simulink model "CompleteCavityModel"  (R2022b)
settings: Solver=VariableStepAuto  StartTime=0.0  StopTime=100  RelTol=1e-3
model workspace (MAT data in the model file):
  KL1 = Simulink.Parameter
  KL1.Value = 0.4
  KL1.DataType = 'auto'
  KL1.Complexity = 'real'
  KL1.Dimensions = [1 1]
  KL2 = Simulink.Parameter
  KL2.Value = 0.3
  KL2.DataType = 'auto'
  KL2.Complexity = 'real'
  KL2.Dimensions = [1 1]
  KL3 = Simulink.Parameter
  KL3.Value = 0.2
  KL3.DataType = 'auto'
  KL3.Complexity = 'real'
  KL3.Dimensions = [1 1]
  QL = Simulink.Parameter
  QL.Value = 960000
  QL.DataType = 'auto'
  QL.Complexity = 'real'
  QL.Dimensions = [1 1]
  Q_k1 = Simulink.Parameter
  Q_k1.Value = 100
  Q_k1.DataType = 'auto'
  Q_k1.Complexity = 'real'
  Q_k1.Dimensions = [1 1]
  Q_k2 = Simulink.Parameter
  Q_k2.Value = 100
  Q_k2.DataType = 'auto'
  Q_k2.Complexity = 'real'
  Q_k2.Dimensions = [1 1]
  Q_k3 = Simulink.Parameter
  Q_k3.Value = 100
  Q_k3.DataType = 'auto'
  Q_k3.Complexity = 'real'
  Q_k3.Dimensions = [1 1]
  RL = Simulink.Parameter
  RL.Value = Simulink.data.Expression
  RL.Value.ExpressionString = "QL*RQ"
  RL.DataType = 'auto'
  RL.Complexity = 'real'
  RL.Dimensions = -1
  RQ = Simulink.Parameter
  RQ.Value = 310
  RQ.DataType = 'auto'
  RQ.Complexity = 'real'
  RQ.Dimensions = [1 1]
  Ts = Simulink.Parameter
  Ts.Value = 1e-10
  Ts.DataType = 'auto'
  Ts.Complexity = 'real'
  Ts.Dimensions = [1 1]
  a0 = Simulink.Parameter
  a0.Value = 1
  a0.DataType = 'auto'
  a0.Complexity = 'real'
  a0.Dimensions = [1 1]
  a1 = Simulink.Parameter
  a1.Value = -2
  a1.DataType = 'auto'
  a1.Complexity = 'real'
  a1.Dimensions = [1 1]
  a2 = Simulink.Parameter
  a2.Value = 1
  a2.DataType = 'auto'
  a2.Complexity = 'real'
  a2.Dimensions = [1 1]
  b0 = Simulink.Parameter
  b0.Value = -2.18e-09
  b0.DataType = 'auto'
  b0.Complexity = 'real'
  b0.Dimensions = [1 1]
  b1 = Simulink.Parameter
  b1.Value = -4.36e-09
  b1.DataType = 'auto'
  b1.Complexity = 'real'
  b1.Dimensions = [1 1]
  b2 = Simulink.Parameter
  b2.Value = -2.18e-09
  b2.DataType = 'auto'
  b2.Complexity = 'real'
  b2.Dimensions = [1 1]
  f0 = Simulink.Parameter
  f0.Value = 648000000
  f0.DataType = 'auto'
  f0.Complexity = 'real'
  f0.Dimensions = [1 1]
  f_k1 = Simulink.Parameter
  f_k1.Value = 235
  f_k1.DataType = 'auto'
  f_k1.Complexity = 'real'
  f_k1.Dimensions = [1 1]
  f_k2 = Simulink.Parameter
  f_k2.Value = 290
  f_k2.DataType = 'auto'
  f_k2.Complexity = 'real'
  f_k2.Dimensions = [1 1]
  f_k3 = Simulink.Parameter
  f_k3.Value = 450
  f_k3.DataType = 'auto'
  f_k3.Complexity = 'real'
  f_k3.Dimensions = [1 1]
  pi = Simulink.Parameter
  pi.Value = 3.1415926535
  pi.DataType = 'auto'
  pi.Complexity = 'real'
  pi.Dimensions = [1 1]
  w0 = Simulink.Parameter
  w0.Value = Simulink.data.Expression
  w0.Value.ExpressionString = "2*pi*390"
  w0.DataType = 'auto'
  w0.Complexity = 'real'
  w0.Dimensions = -1
  w_hbw = Simulink.Parameter
  w_hbw.Value = Simulink.data.Expression
  w_hbw.Value.ExpressionString = "pi*f0/QL"
  w_hbw.DataType = 'auto'
  w_hbw.Complexity = 'real'
  w_hbw.Dimensions = -1
settings Model: Creator=mliu  LastModifiedBy=mliu

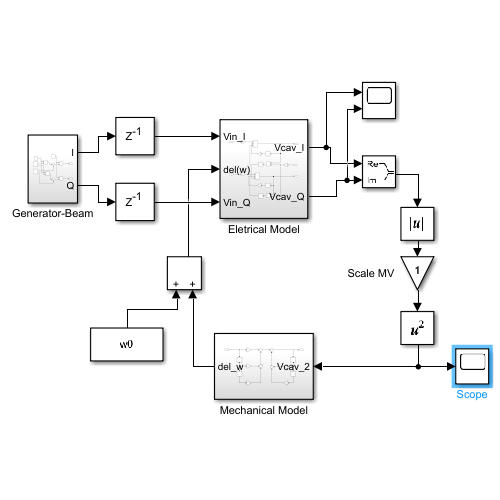
[thumbnail: Simulink's stored preview of the top-level diagram]
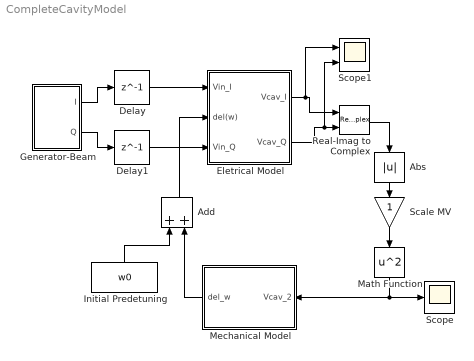
== system CompleteCavityModel ==
  Abs : Abs  SaturateOnIntegerOverflow=off
  Add : Sum
  Delay : Delay  DelayLength=1  InitialCondition=0
  Delay1 : Delay  DelayLength=1  InitialCondition=0
  Eletrical Model : Subsystem
  Generator-Beam : Subsystem
  Initial Predetuning : Constant  Value=w0
  Math Function : Math  Operator=square
  Mechanical Model : Subsystem
  Real-Imag to Complex : RealImagToComplex
  Scale MV : Gain
  Scope : Scope
  Scope1 : Scope  NumInputPorts=2
  wires:
  Delay1/1 -> Eletrical Model/3(Vin_Q)
  Delay/1 -> Eletrical Model/1(Vin_I)
  Eletrical Model/2(Vcav_Q) -> Scope1/2, Real-Imag to Complex/2
  Real-Imag to Complex/1 -> Abs/1
  Abs/1 -> Scale MV/1
  Scale MV/1 -> Math Function/1
  Math Function/1 -> Scope/1, Mechanical Model/1(Vcav_2)
  Add/1 -> Eletrical Model/2(del(w))
  Mechanical Model/1(del_w) -> Add/2
  Initial Predetuning/1 -> Add/1
  Generator-Beam/1(I) -> Delay/1
  Generator-Beam/2(Q) -> Delay1/1
  Eletrical Model/1(Vcav_I) -> Scope1/1, Real-Imag to Complex/1

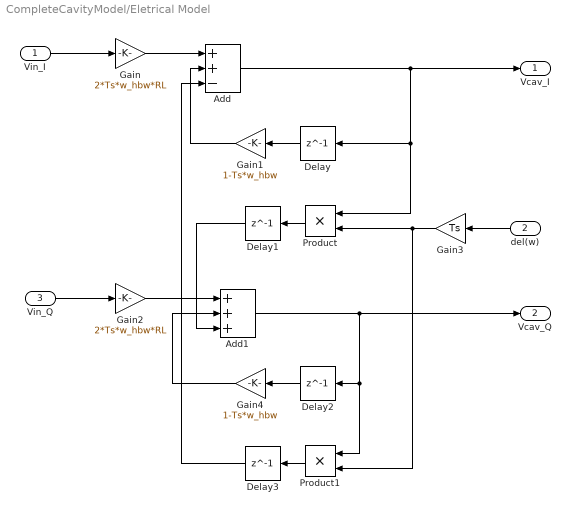
== system CompleteCavityModel/Eletrical Model ==
  Vin_I : Inport
  del(w) : Inport  Port=2
  Vin_Q : Inport  Port=3
  Add : Sum  Inputs=++-
  Add1 : Sum  Inputs=+++
  Delay{,1..3} (4 alike) : Delay  DelayLength=1  InitialCondition=0
  Gain : Gain  Gain=2*Ts*w_hbw*RL
  Gain1 : Gain  Gain=1-Ts*w_hbw
  Gain2 : Gain  Gain=2*Ts*w_hbw*RL
  Gain3 : Gain  Gain=Ts
  Gain4 : Gain  Gain=1-Ts*w_hbw
  Product : Product
  Product1 : Product
  Vcav_I : Outport
  Vcav_Q : Outport  Port=2
  wires:
  Delay/1 -> Gain1/1
  Gain/1 -> Add/1
  Gain3/1 -> Product1/2, Product/2
  Add1/1 -> Vcav_Q/1, Product1/1, Delay2/1
  Add/1 -> Vcav_I/1, Product/1, Delay/1
  Delay1/1 -> Add1/3
  Product/1 -> Delay1/1
  Vin_Q/1 -> Gain2/1
  Vin_I/1 -> Gain/1
  Gain2/1 -> Add1/1
  Product1/1 -> Delay3/1
  Gain1/1 -> Add/2
  Delay2/1 -> Gain4/1
  Delay3/1 -> Add/3
  del(w)/1 -> Gain3/1
  Gain4/1 -> Add1/2

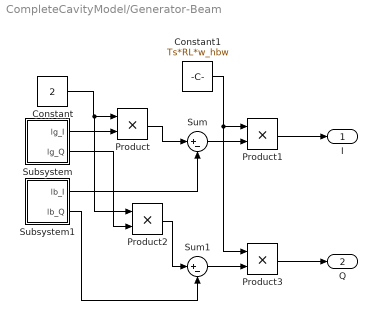
== system CompleteCavityModel/Generator-Beam ==
  Constant : Constant  Value=2
  Constant1 : Constant  Value=Ts*RL*w_hbw
  Product{,1..3} (4 alike) : Product
  Subsystem : Subsystem
  Subsystem1 : Subsystem
  Sum : Sum  Inputs=|+-
  Sum1 : Sum  Inputs=|+-
  I : Outport
  Q : Outport  Port=2
  wires:
  Subsystem1/2(lb_Q) -> Sum1/2
  Constant1/1 -> Product3/1, Product1/1
  Constant/1 -> Product2/1, Product/1
  Product1/1 -> I/1
  Product/1 -> Sum/1
  Subsystem1/1(lb_I) -> Sum/2
  Subsystem/1(lg_I) -> Product/2
  Sum1/1 -> Product3/2
  Product2/1 -> Sum1/1
  Subsystem/2(lg_Q) -> Product2/2
  Sum/1 -> Product1/2
  Product3/1 -> Q/1

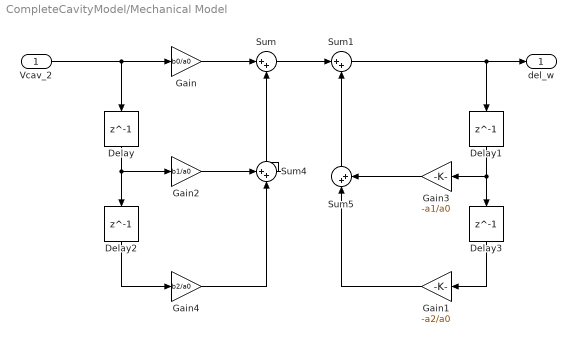
== system CompleteCavityModel/Mechanical Model ==
  Vcav_2 : Inport
  Delay{,1..3} (4 alike) : Delay  DelayLength=1  InitialCondition=0
  Gain : Gain  Gain=b0/a0
  Gain1 : Gain  Gain=-a2/a0
  Gain2 : Gain  Gain=b1/a0
  Gain3 : Gain  Gain=-a1/a0
  Gain4 : Gain  Gain=b2/a0
  Sum{,1,4..5} (4 alike) : Sum  Inputs=|++
  del_w : Outport
  wires:
  Sum5/1 -> Sum1/2
  Gain3/1 -> Sum5/2
  Delay1/1 -> Gain3/1, Delay3/1
  Gain/1 -> Sum/1
  Gain2/1 -> Sum4/1
  Sum1/1 -> del_w/1, Delay1/1
  Sum4/1 -> Sum/2
  Sum/1 -> Sum1/1
  Vcav_2/1 -> Delay/1, Gain/1
  Gain1/1 -> Sum5/1
  Delay2/1 -> Gain4/1
  Gain4/1 -> Sum4/2
  Delay/1 -> Gain2/1, Delay2/1
  Delay3/1 -> Gain1/1

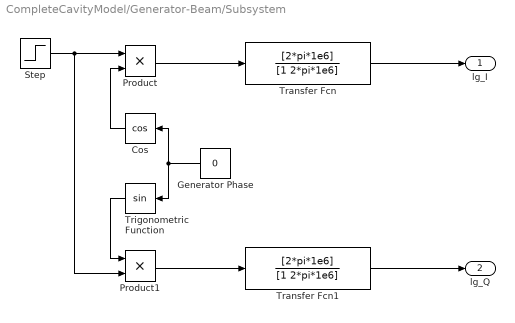
== system CompleteCavityModel/Generator-Beam/Subsystem ==
  Cos : Trigonometry  Operator=cos
  Generator Phase : Constant  Value=0
  Product : Product
  Product1 : Product
  Step : Step  SampleTime=0
  Transfer Fcn : TransferFcn  Numerator=[2*pi*1e6]  Denominator=[1 2*pi*1e6]
  Transfer Fcn1 : TransferFcn  Numerator=[2*pi*1e6]  Denominator=[1 2*pi*1e6]
  Trigonometric Function : Trigonometry
  lg_I : Outport
  lg_Q : Outport  Port=2
  wires:
  Generator Phase/1 -> Trigonometric Function/1, Cos/1
  Transfer Fcn1/1 -> lg_Q/1
  Product1/1 -> Transfer Fcn1/1
  Trigonometric Function/1 -> Product1/1
  Transfer Fcn/1 -> lg_I/1
  Cos/1 -> Product/2
  Product/1 -> Transfer Fcn/1
  Step/1 -> Product1/2, Product/1

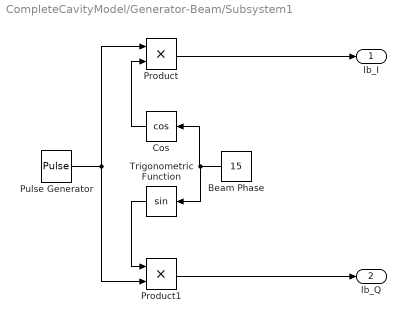
== system CompleteCavityModel/Generator-Beam/Subsystem1 ==
  Beam Phase : Constant  Value=15
  Cos : Trigonometry  Operator=cos
  Product : Product
  Product1 : Product
  Pulse Generator : DiscretePulseGenerator  PulseType=Time based  Period=0.04  PulseWidth=5
  Trigonometric Function : Trigonometry
  lb_I : Outport
  lb_Q : Outport  Port=2
  wires:
  Product/1 -> lb_I/1
  Trigonometric Function/1 -> Product1/1
  Pulse Generator/1 -> Product/1, Product1/2
  Beam Phase/1 -> Trigonometric Function/1, Cos/1
  Product1/1 -> lb_Q/1
  Cos/1 -> Product/2
